simulink model "lazo_cerrado"  (R2018b)
settings: Solver=VariableStepAuto  StartTime=0.0  StopTime=5  RelTol=1e-3
values from neighbouring files (symbols this model uses):
  A = [                        0, 1, 0,                0 ... (first row only)    [sistema.m]
  B = [0; (-L*m*p1)/(M+m); 0; p2]    [sistema.m]
  C = eye(4)    [sistema.m]
  D = zeros(4,1)    [sistema.m]
settings Model: Creator=vuvux  LastModifiedBy=vuvux

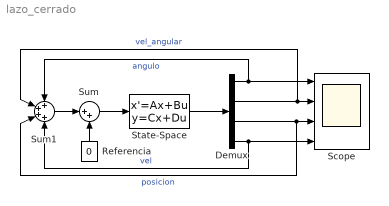
== system lazo_cerrado ==
  Demux : Demux
  Referencia : Constant  Value=0
  Scope : Scope  NumInputPorts=4
  State-Space : StateSpace  A=A  B=B  C=C  D=D  InitialCondition=[2; 0; 0; 0];
  Sum : Sum  Inputs=|++
  Sum1 : Sum  Inputs=++++
  wires:
  State-Space/1 -> Demux/1
  Demux/4 -> Scope/4, Sum1/4  "vel"
  Demux/1 -> Scope/1, Sum1/1  "angulo"
  Demux/2 -> Sum1/2, Scope/2  "vel_angular"
  Demux/3 -> Sum1/3, Scope/3  "posicion"
  Sum/1 -> State-Space/1
  Sum1/1 -> Sum/1
  Referencia/1 -> Sum/2
